simulink model "teste"  (R2025a)
settings: Solver=ode4  StartTime=0.0  StopTime=inf  FixedStep=0.05  RelTol=1e-3  EnableMultiTasking=on
StopFcn:
  | save('dados_da_missao.mat')
undefined symbols (not defined in the file or in its folder): sigbuilder_block
settings Model: Creator=Administrator  LastModifiedBy=Kaue
settings SolverCC: AlgebraicLoopSolver=TrustRegion
settings DataIOCC: LimitDataPoints=on  SaveFormat=StructureWithTime  ReturnWorkspaceOutputs=off
settings OptimizationCC: LifeSpan=inf
settings DebuggingCC: UnconnectedInputMsg=warning  UnconnectedOutputMsg=warning  UnconnectedLineMsg=warning  SFUnexpectedBacktrackingDiag=warning  SFNoUnconditionalDefaultTransitionDiag=warning  SFExecutionAtInitializationDiag=none  ArithmeticOperatorsInVariantConditions=warning
settings HardwareCC: ProdBitPerPointer=32.0  ProdBitPerSizeT=32.0  ProdBitPerPtrDiffT=32.0  ProdLargestAtomicFloat=None  ProdIntDivRoundTo=Undefined  ProdEndianess=Unspecified  ProdWordSize=32.0  ProdHWDeviceType=32-bit Generic
settings ModelReferenceCC: EnableRefExpFcnMdlSchedulingChecks=on  PropagateSignalLabelsOutOfModel=off
settings SFSimCC: SimUseLocalCustomCode=off  CustomCodeUndefinedFunction=UseInterfaceOnly
settings RTWCC: RTWUseLocalCustomCode=off  GPUComputeCapability=3.5
settings CodeAppCC: StateflowObjectComments=on
settings GRTTargetCC: TargetLangStandard=C89/C90 (ANSI)
settings ConfigComp: CovMetricSettings=dw  CovSaveCumulativeToWorkspaceVar=on  CovSaveSingleToWorkspaceVar=on  CovExternalEMLEnable=off

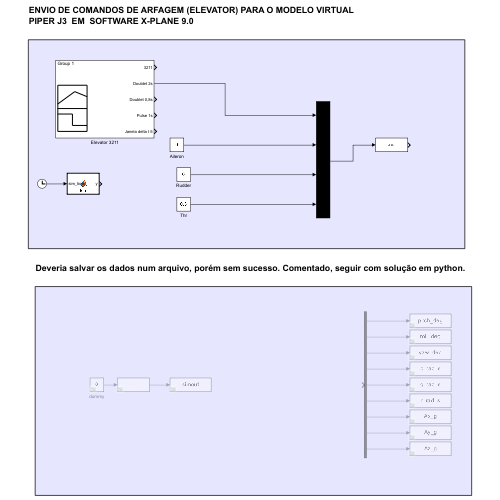
[thumbnail: Simulink's stored preview of the top-level diagram]
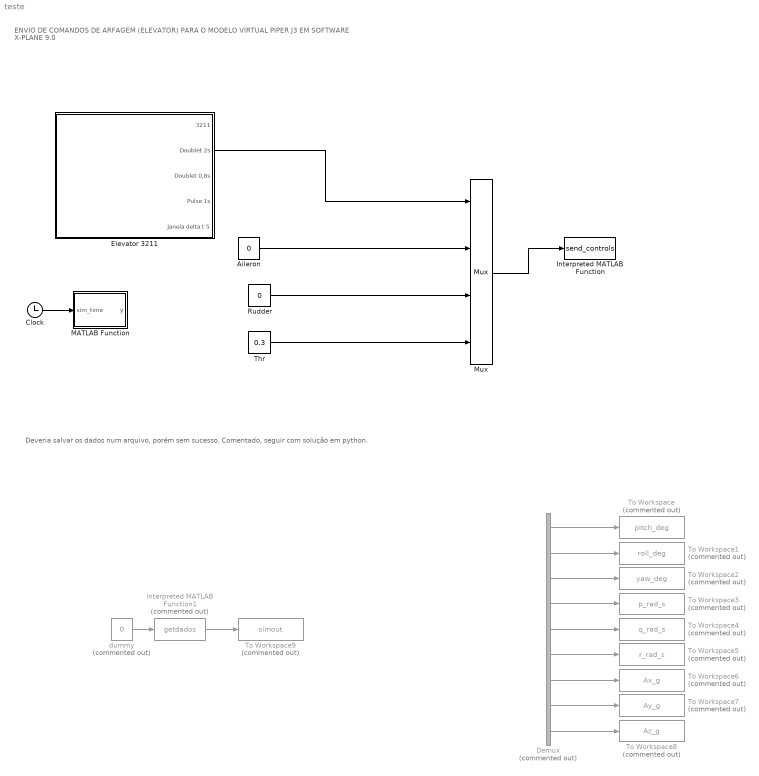
== system teste ==
  note: ENVIO DE COMANDOS DE ARFAGEM (ELEVATOR) PARA O MODELO VIRTUAL
      | PIPER J3 EM SOFTWARE X-PLANE 9.0
  note: Deveria salvar os dados num arquivo, porém sem sucesso. Comentado, seguir com solução em python.
  Aileron : Constant  Value=0
  Clock : Clock
  Demux : Demux  Commented=on  Outputs=9
  Elevator 3211 : Subsystem  Tag=STV Subsys  LoadFcn=sigbuilder_block('load');  StartFcn=sigbuilder_block('start');  StopFcn=sigbuilder_block('stop');  ClipboardFcn=sigbuilder_block('clipboard');  mask(Sigbuilder block){tuvar=[0:10]}
      mask help: Simulink:masks:SigbuilderBlock_MD
      mask init:
      | if ~strcmp(get_param(bdroot(gcbh),'SimulationStatus'),'stopped') tuvar = sigbuilder_block('maskInit'); end
      settings: CopyFcn=sigbuilder_block('copy');  DeleteFcn=sigbuilder_block('delete');  ModelCloseFcn=sigbuilder_block('modelClose');  PreSaveFcn=sigbuilder_block('preSave');  PauseFcn=sigbuilder_block('pause');  ContinueFcn=sigbuilder_block('continue');  NameChangeFcn=sigbuilder_block('namechange');  OpenFcn=sigbuilder_block('open',[437.6 199.2 550.4 400 ]);  CloseFcn=sigbuilder_block('close');
      mask Display: plot(0, 0, 100, 100,[2, 2, 32, 32, 2], [68, 8, 8, 68, 68],[32, 2], [38, 38], [32, 19, 2],[53, 60, 44], [32, 17, 17, 2],[16, 16, 31, 31]);txt = getActiveGroup(gcbh);text(2, 100, txt,'verticalAlignment', 'top');
  Interpreted MATLAB Function : MATLABFcn  MATLABFcn=send_controls
  Interpreted MATLAB Function1 : MATLABFcn  Commented=on  MATLABFcn=getdados  OutputDimensions=9
  MATLAB Function : MATLAB Function  TreatAsAtomicUnit=on
  Mux : Mux
  Rudder : Constant  Value=0
  Thr : Constant  Value=0.3
  To Workspace : ToWorkspace  Commented=on  VariableName=pitch_deg  SaveFormat=Timeseries  SampleTime=-1
  To Workspace1 : ToWorkspace  Commented=on  VariableName=roll_deg  SaveFormat=Timeseries  SampleTime=-1
  To Workspace2 : ToWorkspace  Commented=on  VariableName=yaw_deg  SaveFormat=Timeseries  SampleTime=-1
  To Workspace3 : ToWorkspace  Commented=on  VariableName=p_rad_s  SaveFormat=Timeseries  SampleTime=-1
  To Workspace4 : ToWorkspace  Commented=on  VariableName=q_rad_s  SaveFormat=Timeseries  SampleTime=-1
  To Workspace5 : ToWorkspace  Commented=on  VariableName=r_rad_s  SaveFormat=Timeseries  SampleTime=-1
  To Workspace6 : ToWorkspace  Commented=on  VariableName=Ax_g  SaveFormat=Timeseries  SampleTime=-1
  To Workspace7 : ToWorkspace  Commented=on  VariableName=Ay_g  SaveFormat=Timeseries  SampleTime=-1
  To Workspace8 : ToWorkspace  Commented=on  VariableName=Az_g  SaveFormat=Timeseries  SampleTime=-1
  To Workspace9 : ToWorkspace  Commented=on  VariableName=simout  SaveFormat=Timeseries  SampleTime=-1
  dummy : Constant  Commented=on  Value=0
  wires:
  Rudder/1 -> Mux/3
  Thr/1 -> Mux/4
  Mux/1 -> Interpreted MATLAB Function/1
  Aileron/1 -> Mux/2
  dummy/1 -> Interpreted MATLAB Function1/1
  Demux/1 -> To Workspace/1
  Demux/2 -> To Workspace1/1
  Demux/3 -> To Workspace2/1
  Demux/4 -> To Workspace3/1
  Demux/5 -> To Workspace4/1
  Demux/6 -> To Workspace5/1
  Demux/7 -> To Workspace6/1
  Demux/8 -> To Workspace7/1
  Demux/9 -> To Workspace8/1
  Interpreted MATLAB Function1/1 -> To Workspace9/1
  Clock/1 -> MATLAB Function/1(sim_time)
  Elevator 3211/2(Doublet 2s) -> Mux/1

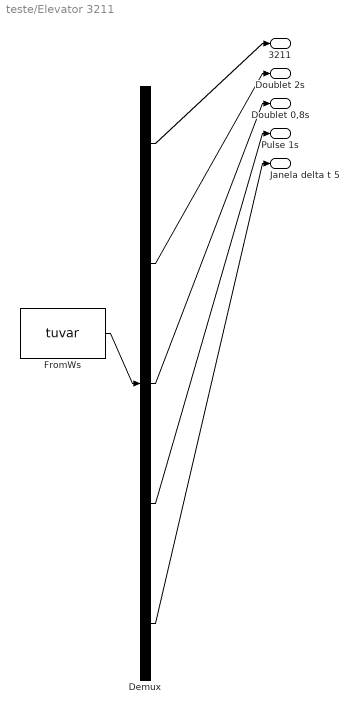
== system teste/Elevator 3211 ==
  Demux : Demux  Tag=STV Demux  Outputs=5
      settings: DisplayOption=none
  FromWs : FromWorkspace  Tag=STV FromWs  VariableName=tuvar
      SigBuilderData=|
      | common.afterFinalStr = 'Extrapolate'
      | common.sampleTime = '0'
      | dataSet.timeRange = [0 100]
      | dataSet.name = 'Group 1'
      | sbobj.Groups.Name = 'Group 1'
      | sbobj.Groups.Signals(1).Name = '3211'
      | sbobj.Groups.Signals(1).XData = [0 5 5 5.1 5.2 8 8 10 10 11 11 12 12 100]
      | sbobj.Groups.Signals(1).YData = [0 0 0.2 0.2 0.2 0.2 -0.2 -0.2 0.2 0.2 -0.2 -0.2 0 0]
      | sbobj.Groups.Signals(2).Name = 'Doublet 2s'
      | sbobj.Groups.Signals(2).XData = [0 5 5 6 6 7 7 100]
      | sbobj.Groups.Signals(2).YData = [0 0 0.2 0.2 -0.198 -0.198 0 0]
      | sbobj.Groups.Signals(3).Name = 'Doublet 0,8s'
      | sbobj.Groups.Signals(3).XData = [0 5 5 5.4 5.4 5.8 5.8 100]
      | sbobj.Groups.Signals(3).YData = [0 0 0.2 0.2 -0.198 -0.198 0 0]
      | sbobj.Groups.Signals(4).Name = 'Pulse 1s'
      | sbobj.Groups.Signals(4).XData = [0 5 5 6 6 100]
      | sbobj.Groups.Signals(4).YData = [0 0 0.2 0.2 0 0]
      | sbobj.Groups.Signals(5).Name = 'Janela delta t 5'
      | sbobj.Groups.Signals(5).XData = [0 0.1 0.2 0.3 0.4 0.5 0.6 0.7 0.8 0.9 1 1.1 1.2 1.3 1.4 1.5 1.6 1.7 1.8 1.9 2 2.1 2.2 2.3 2.4 2.5 2.6 2.7 2.8 2.9 3 3.1 3.2 3.3 3.4 3.5 3.6 3.7 3.8 3.9 4 4.1 4.2 4.3 4.4 4.5 4.6 4.7 4.8 4.9 5 5.1 5.2 5.3 5.4 5.5 5.6 5.7 5.8 5.9 6 6.1 6.2 6.3 6.4 6.5 6.6 6.7 6.8 6.9 7 7.1 7.2 7.3 7.4 7.5 7.6 7.7 7.8 7.9 8 8.1 8.2 8.3 8.4 8.5 8.6 8.7 8.8 8.9 9 9.1 9.2 9.3 9.4 9.5 9.6 9.7 9.8 9.9 100]
      | sbobj.Groups.Signals(5).YData = [0.0196349540849 0.0196349540849 0.0196349540849 0.0194643599637 0.0116817814396 0.00765518966713 0.0169049757658 0.018891454736 0.0196349540849 0.0196349540849 0.0196349540849 0.0196349540849 0.0196349540849 0.0196349540849 0.0179523574034 0.0191731785037 0.0196349540849 0.0196349540849 0.0196349540849 0.0196349540849 0.0196349540849 0.0196349540849 0.0314787404534 0.0839220028003 0.198297815363 0.188959503412 0.0178814932476 -0.25870342875 -0.118169654383 0.0196349540849 0.0196349540849 0.0196349540849 0.0196349540849 0.0196349540849 0.0196349540849 0.0196349540849 0.0196349540849 0.0196349540849 0.0196349540849 0.0196349540849 0.0196349540849 0.0196349540849 0.0196349540849 0.0196349540849 0.0196349540849 0.0196349540849 0.0196349540849 0.0196349540849 0.0196349540849 0.0196349540849 0.0196349540849 0.0196349540849 0.0196349540849 0.0196349540849 0.0196349540849 0.0196349540849 0.0196349540849 0.0196349540849 0.0196349540849 0.0196349540849 0.0196349540849 0.0196349540849 0.0196349540849 0.0196349540849 0.0196349540849 0.0196349540849 0.0196349540849 0.0196349540849 0.0196349540849 0.0196349540849 0.0196349540849 0.0196349540849 0.0196349540849 0.0196349540849 0.0196349540849 0.0196349540849 0.0196349540849 0.0196349540849 0.0196349540849 0.0196349540849 0.0196349540849 0.0196349540849 0.0196349540849 0.0196349540849 0.0196349540849 0.0196349540849 0.0196349540849 0.0218905135147 0.0271099036102 0.0301069295969 0.0311266271794 0.0327616225817 0.0340801153602 0.0403792423468 0.0492883514228 0.051799395427 0.0504916604523 0.0493694755119 0.034098029423 0.0237390701567 0.0237390701567]
      | sbobj.Groups.TimeRange = [0 100]
  3211 : Outport  Tag=STV Outport
  Doublet 2s : Outport  Tag=STV Outport  Port=2
  Doublet 0,8s : Outport  Tag=STV Outport  Port=3
  Pulse 1s : Outport  Tag=STV Outport  Port=4
  Janela delta t 5 : Outport  Tag=STV Outport  Port=5
  wires:
  FromWs/1 -> Demux/1
  Demux/1 -> 3211/1
  Demux/2 -> Doublet 2s/1
  Demux/3 -> Doublet 0,8s/1
  Demux/4 -> Pulse 1s/1
  Demux/5 -> Janela delta t 5/1

== matlab function teste/MATLAB Function ==
  data: sim_time input; y output
function y = fcn(sim_time)
% Este bloco força a simulação do Simulink a rodar em sincronia com o tempo real.

% Variáveis persistentes mantêm seu valor entre as chamadas da função
persistent last_tic
persistent first_step

% Inicialização no primeiro passo da simulação
if isempty(first_step)
    last_tic = tic;      % Inicia o cronômetro de alta precisão
    first_step = false;  % Marca que a inicialização já ocorreu
end

% Tempo real que passou desde a última execução deste bloco
elapsed_real_time = toc(last_tic);

% Tempo de simulação que deveria ter passado (dado pela entrada do bloco)
% Assumimos que a simulação começa em t=0
elapsed_sim_time = sim_time;

% Se o tempo real for menor que o tempo da simulação, a simulação está adiantada.
% Precisamos pausar para esperar o tempo real "alcançar".
if elapsed_real_time < elapsed_sim_time
    pause_duration = elapsed_sim_time - elapsed_real_time;
    pause(pause_duration);
end

% A saída do bloco não é usada, mas é necessária
y = 0;

% Atualiza o cronômetro para o próximo passo (opcional, mas pode ser mais robusto)
% last_tic = tic; % Descomente esta linha para resetar o cronômetro a cada passo

end
